simulink model "Trajectorygenerator_ComputedTorque"  (R2017b)
settings: Solver=ode2  StartTime=0.0  StopTime=12  FixedStep=0.001  RelTol=1e-3
values from neighbouring files (symbols this model uses):
  joint1_initial_deg = 0    [Preload.m]    (also in PreloadTest.m = 25)
  joint2_initial_deg = 0    [Preload.m]    (also in PreloadTest.m = 70)
  joint3_initial_deg = -25    [Preload.m]    (also in PreloadTest.m = 60)
  joint4_initial_deg = 90    [Preload.m]    (also in PreloadTest.m = 20)
  joint5_initial_deg = 0    [Preload.m]    (also in PreloadTest.m = 22)
  joint6_initial_deg = 90    [Preload.m]    (also in PreloadTest.m = 60)
  joint7_initial_deg = 0    [Preload.m]    (also in PreloadTest.m = 30)
  kuk = SerialLink(L)    [Preload.m]    (also in PreloadTest.m)
  qpose = [joint1_initial_deg,joint2_initial_deg,joint3_initial_deg,joint4_initial_deg,joint5_initial_deg,joint6_initial_deg,joint7_initial_deg]*pi/180    [Preload.m]    (also in PreloadTest.m = [joint1_initial_deg,joint2_initial_deg,joint3_initial_deg,jo; onelinkrobotnamedbob.m = [j1_init]; threelinkrobotnamedbob.m = [j1_init j2_init j3_init])
undefined symbols (not defined in the file or in its folder): jacky
settings Model: Creator=mkiri  LastModifiedBy=mkiri

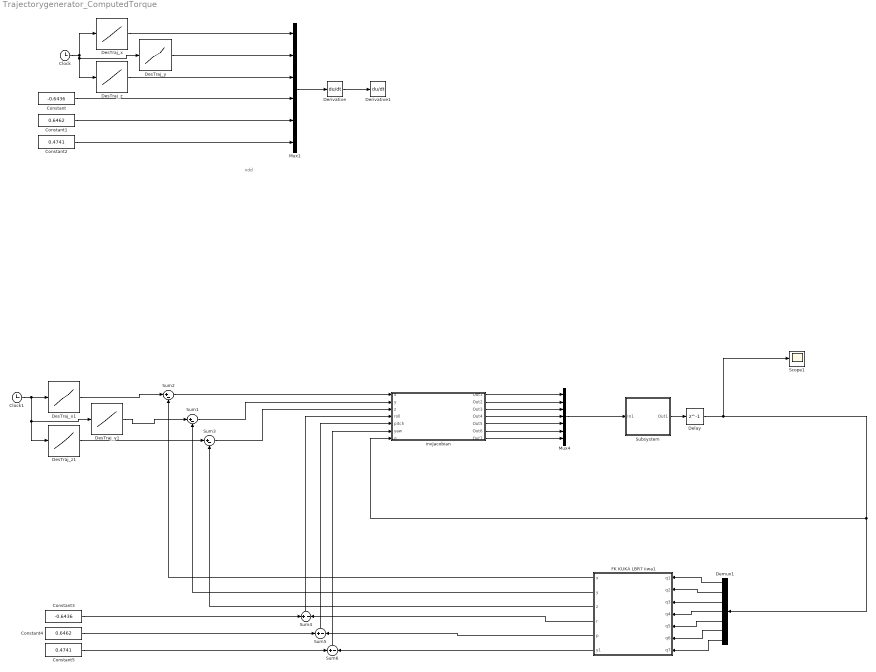
== system Trajectorygenerator_ComputedTorque ==
  note: xdd
  Clock : Clock
  Clock1 : Clock
  Constant : Constant  Value=-0.6436
  Constant1 : Constant  Value=0.6462
  Constant2 : Constant  Value=0.4741
  Constant3 : Constant  Value=-0.6436
  Constant4 : Constant  Value=0.6462
  Constant5 : Constant  Value=0.4741
  Delay : Delay  DelayLength=1  InitialCondition=qpose
  Demux1 : Demux  Outputs=7
  Derivative : Derivative
  Derivative1 : Derivative
  DesTraj_x : Lookup_n-D  NumberOfTableDimensions=1  BreakpointsForDimension1=[0 5]  Table=[0.2314 0.2314]  ExtrapMethod=Clip  UseLastTableValue=on  InternalRulePriority=Speed  RndMeth=Simplest  InputSameDT=on
  DesTraj_x1 : Lookup_n-D  NumberOfTableDimensions=1  BreakpointsForDimension1=[0 5]  Table=[0.2314 0.2314]  ExtrapMethod=Clip  UseLastTableValue=on  InternalRulePriority=Speed  RndMeth=Simplest  InputSameDT=on
  DesTraj_y : Lookup_n-D  NumberOfTableDimensions=1  BreakpointsForDimension1=[0 12]  Table=[-0.2689 0.0689]  ExtrapMethod=Clip  UseLastTableValue=on  InternalRulePriority=Speed  RndMeth=Simplest  InputSameDT=on
  DesTraj_y1 : Lookup_n-D  NumberOfTableDimensions=1  BreakpointsForDimension1=[0 12]  Table=[-0.2689 0.0689]  ExtrapMethod=Clip  UseLastTableValue=on  InternalRulePriority=Speed  RndMeth=Simplest  InputSameDT=on
  DesTraj_z : Lookup_n-D  NumberOfTableDimensions=1  BreakpointsForDimension1=[0 3 6 9 12]  Table=[0.9093 0.7093 0.9093 0.7093 0.9093]  InterpMethod=Cubic spline  ExtrapMethod=Clip  UseLastTableValue=on  InternalRulePriority=Speed  RndMeth=Simplest  InputSameDT=on
  DesTraj_z1 : Lookup_n-D  NumberOfTableDimensions=1  BreakpointsForDimension1=[0 3 6 9 12]  Table=[0.9093 0.7093 0.9093 0.7093 0.9093]  InterpMethod=Cubic spline  ExtrapMethod=Clip  UseLastTableValue=on  InternalRulePriority=Speed  RndMeth=Simplest  InputSameDT=on
  FK KUKA LBR7 iiwa1 : MATLAB Function  TreatAsAtomicUnit=on
  Mux1 : Mux  Inputs=6
  Mux4 : Mux  Inputs=7
  Scope1 : Scope
  Subsystem : Subsystem
  Sum1 : Sum  Inputs=|+-
  Sum2 : Sum  Inputs=|+-
  Sum3 : Sum  Inputs=|+-
  Sum4 : Sum  Inputs=+-
  Sum5 : Sum  Inputs=+-
  Sum6 : Sum  Inputs=+-
  invJacobian : Subsystem
  wires:
  Clock/1 -> DesTraj_y/1, DesTraj_z/1, DesTraj_x/1
  DesTraj_y/1 -> Mux1/2
  DesTraj_x/1 -> Mux1/1
  DesTraj_z/1 -> Mux1/3
  Mux1/1 -> Derivative/1
  Constant1/1 -> Mux1/5
  Constant2/1 -> Mux1/6
  Constant/1 -> Mux1/4
  Derivative/1 -> Derivative1/1
  invJacobian/1(Out1) -> Mux4/1
  invJacobian/7(Out7) -> Mux4/7
  invJacobian/4(Out4) -> Mux4/4
  invJacobian/3(Out3) -> Mux4/3
  invJacobian/2(Out2) -> Mux4/2
  invJacobian/5(Out5) -> Mux4/5
  Constant4/1 -> Sum5/1
  Sum3/1 -> invJacobian/3(z)
  Subsystem/1(Out1) -> Delay/1
  FK KUKA LBR7 iiwa1/3(z) -> Sum3/2
  Constant3/1 -> Sum4/1
  Sum5/1 -> invJacobian/5(pitch)
  Demux1/7 -> FK KUKA LBR7 iiwa1/7(q7)
  FK KUKA LBR7 iiwa1/6(y1) -> Sum6/2
  FK KUKA LBR7 iiwa1/5(p) -> Sum5/2
  FK KUKA LBR7 iiwa1/1(x) -> Sum2/2
  Demux1/3 -> FK KUKA LBR7 iiwa1/3(q3)
  Demux1/4 -> FK KUKA LBR7 iiwa1/4(q4)
  Demux1/1 -> FK KUKA LBR7 iiwa1/1(q1)
  Demux1/5 -> FK KUKA LBR7 iiwa1/5(q5)
  Demux1/2 -> FK KUKA LBR7 iiwa1/2(q2)
  FK KUKA LBR7 iiwa1/4(r) -> Sum4/2
  Sum6/1 -> invJacobian/6(yaw)
  Sum2/1 -> invJacobian/1(x)
  Sum4/1 -> invJacobian/4(roll)
  Clock1/1 -> DesTraj_y1/1, DesTraj_z1/1, DesTraj_x1/1
  Mux4/1 -> Subsystem/1(In1)
  Sum1/1 -> invJacobian/2(y)
  DesTraj_x1/1 -> Sum2/1
  Constant5/1 -> Sum6/1
  invJacobian/6(Out6) -> Mux4/6
  Delay/1 -> Scope1/1, Demux1/1, invJacobian/7(q)
  DesTraj_z1/1 -> Sum3/1
  DesTraj_y1/1 -> Sum1/1
  Demux1/6 -> FK KUKA LBR7 iiwa1/6(q6)
  FK KUKA LBR7 iiwa1/2(y) -> Sum1/2

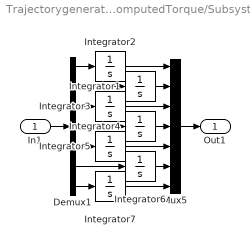
== system Trajectorygenerator_ComputedTorque/Subsystem ==
  In1 : Inport
  Demux1 : Demux  Outputs=7
  Integrator1 : Integrator  InitialCondition=joint2_initial_deg*pi/180
  Integrator2 : Integrator  InitialCondition=joint1_initial_deg*pi/180
  Integrator3 : Integrator  InitialCondition=joint3_initial_deg*pi/180
  Integrator4 : Integrator  InitialCondition=joint4_initial_deg*pi/180
  Integrator5 : Integrator  InitialCondition=joint5_initial_deg*pi/180
  Integrator6 : Integrator  InitialCondition=joint6_initial_deg*pi/180
  Integrator7 : Integrator  InitialCondition=joint7_initial_deg*pi/180
  Mux5 : Mux  Inputs=7
  Out1 : Outport
  wires:
  In1/1 -> Demux1/1
  Mux5/1 -> Out1/1
  Demux1/1 -> Integrator2/1
  Demux1/2 -> Integrator1/1
  Demux1/6 -> Integrator6/1
  Demux1/5 -> Integrator5/1
  Integrator5/1 -> Mux5/5
  Demux1/4 -> Integrator4/1
  Integrator7/1 -> Mux5/7
  Integrator1/1 -> Mux5/2
  Integrator4/1 -> Mux5/4
  Demux1/3 -> Integrator3/1
  Integrator2/1 -> Mux5/1
  Integrator6/1 -> Mux5/6
  Demux1/7 -> Integrator7/1
  Integrator3/1 -> Mux5/3

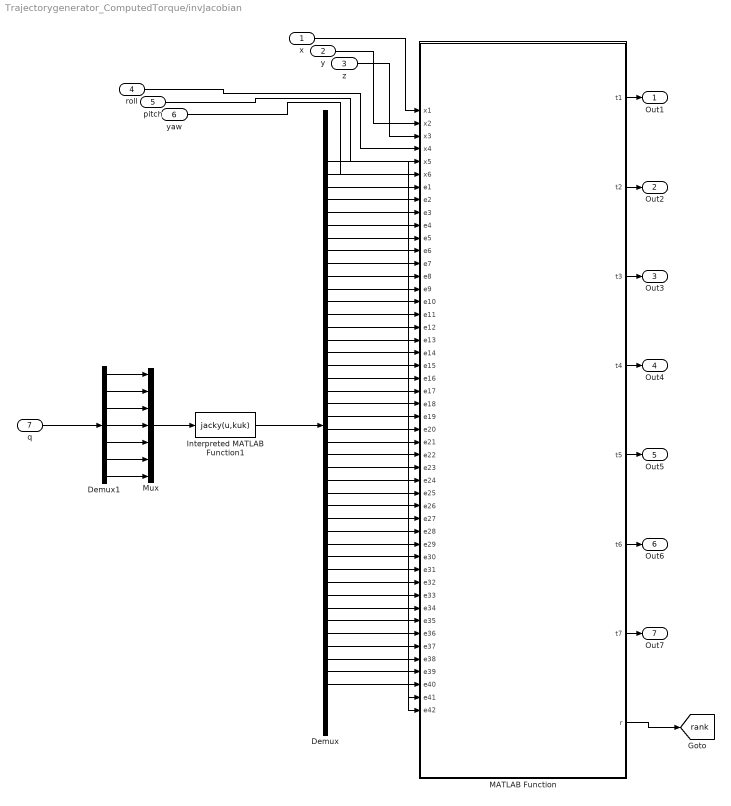
== system Trajectorygenerator_ComputedTorque/invJacobian ==
  x : Inport
  y : Inport  Port=2
  z : Inport  Port=3
  roll : Inport  Port=4
  pitch : Inport  Port=5
  yaw : Inport  Port=6
  q : Inport  Port=7
  Demux : Demux  Outputs=42
  Demux1 : Demux  Outputs=7
  Interpreted MATLAB Function1 : MATLABFcn  MATLABFcn=jacky(u,kuk)
  MATLAB Function : MATLAB Function  TreatAsAtomicUnit=on
  Mux : Mux  Inputs=7
  Out1 : Outport
  Out2 : Outport  Port=2
  Out3 : Outport  Port=3
  Out4 : Outport  Port=4
  Out5 : Outport  Port=5
  Out6 : Outport  Port=6
  Out7 : Outport  Port=7
  tag scope: rank=global
  wires:
  x/1 -> MATLAB Function/1(x1)
  MATLAB Function/2(t2) -> Out2/1
  MATLAB Function/3(t3) -> Out3/1
  y/1 -> MATLAB Function/2(x2)
  MATLAB Function/1(t1) -> Out1/1
  MATLAB Function/4(t4) -> Out4/1
  MATLAB Function/5(t5) -> Out5/1
  z/1 -> MATLAB Function/3(x3)
  MATLAB Function/7(t7) -> Out7/1
  MATLAB Function/6(t6) -> Out6/1
  Interpreted MATLAB Function1/1 -> Demux/1
  Demux/17 -> MATLAB Function/23(e17)
  Demux/16 -> MATLAB Function/22(e16)
  Demux/15 -> MATLAB Function/21(e15)
  Demux/19 -> MATLAB Function/25(e19)
  Demux/14 -> MATLAB Function/20(e14)
  Demux/13 -> MATLAB Function/19(e13)
  Demux/18 -> MATLAB Function/24(e18)
  Demux/20 -> MATLAB Function/26(e20)
  Demux/21 -> MATLAB Function/27(e21)
  Demux/12 -> MATLAB Function/18(e12)
  Demux/6 -> MATLAB Function/12(e6)
  Demux/28 -> MATLAB Function/34(e28)
  Demux/23 -> MATLAB Function/29(e23)
  Demux/5 -> MATLAB Function/11(e5)
  Demux/25 -> MATLAB Function/31(e25)
  Demux/22 -> MATLAB Function/28(e22)
  Demux/9 -> MATLAB Function/15(e9)
  Demux/10 -> MATLAB Function/16(e10)
  Demux/7 -> MATLAB Function/13(e7)
  Demux/11 -> MATLAB Function/17(e11)
  Demux/8 -> MATLAB Function/14(e8)
  Demux/27 -> MATLAB Function/33(e27)
  Demux/26 -> MATLAB Function/32(e26)
  Demux/24 -> MATLAB Function/30(e24)
  Demux/3 -> MATLAB Function/9(e3)
  Demux/38 -> MATLAB Function/44(e38)
  Demux/33 -> MATLAB Function/39(e33)
  Demux/39 -> MATLAB Function/45(e39)
  Demux/36 -> MATLAB Function/42(e36)
  Demux/41 -> MATLAB Function/47(e41)
  Demux/42 -> MATLAB Function/48(e42)
  Demux/40 -> MATLAB Function/46(e40)
  Demux/34 -> MATLAB Function/40(e34)
  Demux/31 -> MATLAB Function/37(e31)
  Demux/30 -> MATLAB Function/36(e30)
  Demux/2 -> MATLAB Function/8(e2)
  Demux/4 -> MATLAB Function/10(e4)
  Demux/32 -> MATLAB Function/38(e32)
  Demux/1 -> MATLAB Function/7(e1)
  Demux/35 -> MATLAB Function/41(e35)
  Demux/37 -> MATLAB Function/43(e37)
  Demux/29 -> MATLAB Function/35(e29)
  q/1 -> Demux1/1
  Demux1/3 -> Mux/3
  Demux1/2 -> Mux/2
  Demux1/4 -> Mux/4
  Demux1/1 -> Mux/1
  Demux1/5 -> Mux/5
  Demux1/6 -> Mux/6
  Demux1/7 -> Mux/7
  Mux/1 -> Interpreted MATLAB Function1/1
  yaw/1 -> MATLAB Function/6(x6)
  pitch/1 -> MATLAB Function/5(x5)
  roll/1 -> MATLAB Function/4(x4)
  MATLAB Function/8(r) -> [rank]

== matlab function Trajectorygenerator_ComputedTorque/invJacobian/MATLAB Function ==
  data: x1 input; t1 output; x2 input; x3 input; x4 input; x5 input; x6 input; e1 input; e2 input; e3 input; e4 input; e5 input; e6 input; e7 input; e8 input; e9 input; e10 input; e11 input; e12 input; e13 input; e14 input; e15 input; e16 input; e17 input; e18 input; e19 input; e20 input; e21 input; e22 input; e23 input; e24 input; e25 input; e26 input; e27 input; e28 input; e29 input; e30 input; e31 input; e32 input; e33 input; e34 input; e35 input; e36 input; e37 input; e38 input; e39 input; e40 input; e41 input; e42 input; t2 output; t3 output; t4 output; t5 output; t6 output; t7 output; r output
function [t1,t2,t3,t4,t5,t6,t7,r] = fcn(x1,x2,x3,x4,x5,x6,e1,e2,e3,e4,e5,e6,e7,e8,e9,e10,e11,e12,e13,e14,e15,e16,e17,e18,e19,e20,e21,e22,e23,e24,e25,e26,e27,e28,e29,e30,e31,e32,e33,e34,e35,e36,e37,e38,e39,e40,e41,e42)

J = [e1	e7	e13	e19	e25	e31	e37
e2	e8	e14	e20	e26	e32	e38
e3	e9	e15	e21	e27	e33	e39
e4	e10	e16	e22	e28	e34	e40
e5	e11	e17	e23	e29	e35	e41
e6	e12	e18	e24	e30	e36	e42];
X = [x1;x2;x3;x4;x5;x6];
%Js = J((1):(3),(1):(7));
Js = J;
Q = pinv(Js)*X;

t1 = Q(1,:);
t2 = Q(2,:);
t3 = Q(3,:);
t4 = Q(4,:);
t5 = Q(5,:);
t6 = Q(6,:);
t7 = Q(7,:);
r = rank(Js);

== matlab function Trajectorygenerator_ComputedTorque/FK KUKA LBR7 iiwa1 ==
  data: x output; q1 input; y output; q2 input; q3 input; q4 input; q5 input; q6 input; q7 input; z output; r output; p output; y1 output
function [x,y,z,r,p,y1] = fcn(q1,q2,q3,q4,q5,q6,q7)
T1 = [cos(q1),0,sin(q1),0;sin(q1),0,(-1)*cos(q1),0;0,1,0,0.34E0;0,0,0, ...
1];
T2 = [cos(q2),0,(-1)*sin(q2),0;sin(q2),0,cos(q2),0;0,(-1),0,0;0,0,0, ...
  1];
T3 = [cos(q3),0,(-1)*sin(q3),0;sin(q3),0,cos(q3),0;0,(-1),0,0.4E0;0,0, ...
  0,1];
T4 = [cos(q4),0,sin(q4),0;sin(q4),0,(-1)*cos(q4),0;0,1,0,0;0,0,0,1];
T5 = [cos(q5),0,sin(q5),0;sin(q5),0,(-1)*cos(q5),0;0,1,0,0.4E0;0,0,0, ...
  1];
T6 = [cos(q6),0,(-1)*sin(q6),0;sin(q6),0,cos(q6),0;0,(-1),0,0;0,0,0, ...
  1];
T7 = [cos(q7),0,sin(q7),0;sin(q7),0,(-1)*cos(q7),0;0,1,0,0.126E0;0,0, ...
  0,1];

T = T1*T2*T3*T4*T5*T6*T7;

x=T(1,4);
y=(T(2,4));
z=T(3,4);
r = atan(T(3,2)/T(3,3));
p = atan(-1*T(3,1)/sqrt((T(3,2))^2+(T(3,3))^2));
y1 = atan(T(2,1)/T(1,1));
